simulink model "atril_v2"  (R2019a)
settings: Solver=VariableStepAuto  StartTime=0.0  StopTime=inf  RelTol=1e-3
settings Model: Creator=ASUS  LastModifiedBy=mateo

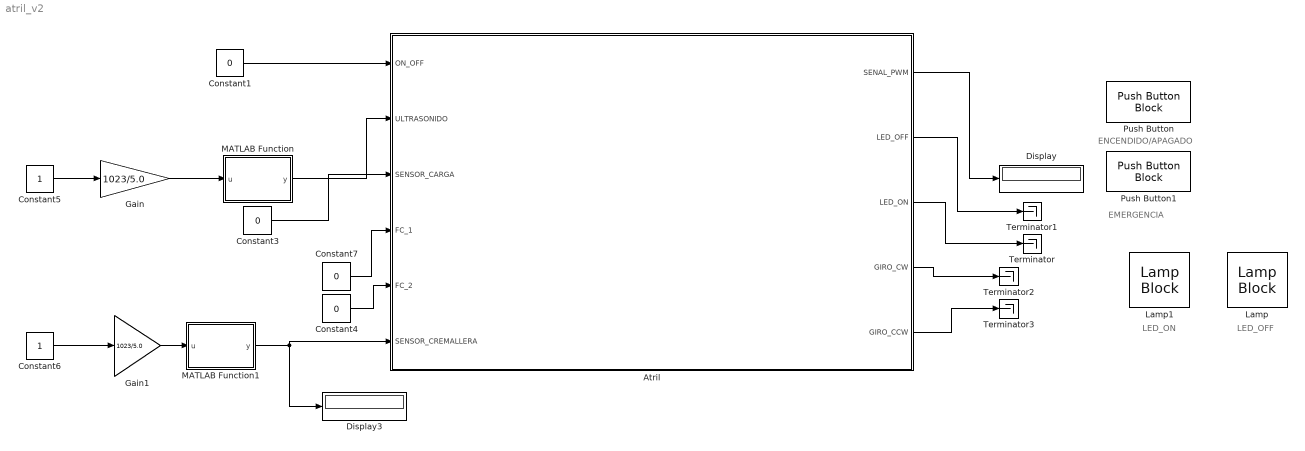
== system atril_v2 ==
  note: LED_OFF
  note: LED_ON
  note: ENCENDIDO/APAGADO
  note: EMERGENCIA
  Atril : Subsystem
  Constant{1,3..4,7} (4 alike) : Constant  Value=0
  Constant5 : Constant
  Constant6 : Constant
  Display : Display
  Display3 : Display
  Gain : Gain  Gain=1023/5.0
  Gain1 : Gain  Gain=1023/5.0
  Lamp : LampBlock  WebBlockId=10
  Lamp1 : LampBlock  WebBlockId=11
  MATLAB Function : MATLAB Function  TreatAsAtomicUnit=on
  MATLAB Function1 : MATLAB Function  TreatAsAtomicUnit=on
  Push Button : PushButtonBlock  WebBlockId=25
  Push Button1 : PushButtonBlock  WebBlockId=26
  Terminator{,1..3} (4 alike) : Terminator
  wires:
  Gain1/1 -> MATLAB Function1/1(u)
  Constant6/1 -> Gain1/1
  Constant5/1 -> Gain/1
  Gain/1 -> MATLAB Function/1(u)
  MATLAB Function1/1(y) -> Atril/6(SENSOR_CREMALLERA), Display3/1
  Constant1/1 -> Atril/1(ON_OFF)
  MATLAB Function/1(y) -> Atril/2(ULTRASONIDO)
  Constant3/1 -> Atril/3(SENSOR_CARGA)
  Constant7/1 -> Atril/4(FC_1)
  Constant4/1 -> Atril/5(FC_2)
  Atril/1(SENAL_PWM) -> Display/1
  Atril/2(LED_OFF) -> Terminator1/1
  Atril/3(LED_ON) -> Terminator/1
  Atril/4(GIRO_CW) -> Terminator2/1
  Atril/5(GIRO_CCW) -> Terminator3/1

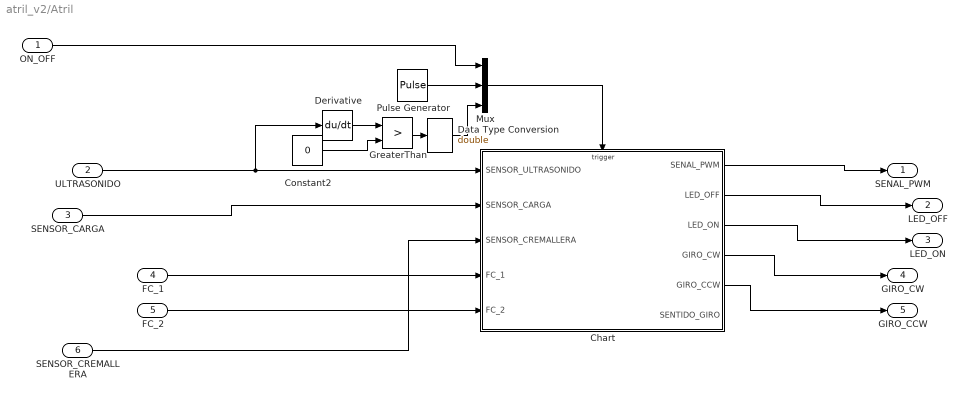
== system atril_v2/Atril ==
  ON_OFF : Inport
  ULTRASONIDO : Inport  Port=2
  SENSOR_CARGA : Inport  Port=3
  FC_1 : Inport  Port=4
  FC_2 : Inport  Port=5
  SENSOR_CREMALLERA : Inport  Port=6
  Chart : Stateflow chart  TreatAsAtomicUnit=on
  Constant2 : Constant  Value=0
  Data Type Conversion : DataTypeConversion  OutDataTypeStr=double
  Derivative : Derivative
  GreaterThan : RelationalOperator  Operator=>  OutDataTypeStr=boolean  RndMeth=Simplest
  Mux : Mux  Inputs=3
  Pulse Generator : DiscretePulseGenerator  PulseType=Time based  Period=10  PulseWidth=0.5
  SENAL_PWM : Outport
  LED_OFF : Outport  Port=2
  LED_ON : Outport  Port=3
  GIRO_CW : Outport  Port=4
  GIRO_CCW : Outport  Port=5
  wires:
  Pulse Generator/1 -> Mux/2
  Constant2/1 -> GreaterThan/2
  ULTRASONIDO/1 -> Chart/1(SENSOR_ULTRASONIDO), Derivative/1
  Mux/1 -> Chart/Trigger
  SENSOR_CREMALLERA/1 -> Chart/3(SENSOR_CREMALLERA)
  SENSOR_CARGA/1 -> Chart/2(SENSOR_CARGA)
  ON_OFF/1 -> Mux/1
  Derivative/1 -> GreaterThan/1
  Chart/1(SENAL_PWM) -> SENAL_PWM/1
  FC_2/1 -> Chart/5(FC_2)
  Chart/2(LED_OFF) -> LED_OFF/1
  FC_1/1 -> Chart/4(FC_1)
  Chart/3(LED_ON) -> LED_ON/1
  Chart/4(GIRO_CW) -> GIRO_CW/1
  Chart/5(GIRO_CCW) -> GIRO_CCW/1
  GreaterThan/1 -> Data Type Conversion/1
  Data Type Conversion/1 -> Mux/3

== matlab function atril_v2/MATLAB Function1 ==
  data: u input; y output
function y = fcn(u)

y = u;

== matlab function atril_v2/MATLAB Function ==
  data: u input; y output
function y = fcn(u)

y = u;

== stateflow chart atril_v2/Atril/Chart ==
  state ESTADO_ON
    state e1
      entry:
      LED_ON=1;
      LED_OFF=0;
      SENAL_PWM=0;
      SENTIDO_GIRO=0;
    state Stand_by
    state e4
      entry:
      SENAL_PWM=0.5;
      GIRO_CW=0;
      GIRO_CCW=1;
    state e2
      entry:
      SENAL_PWM=0.5;
      GIRO_CW=1;
      GIRO_CCW=0;
      FC=SENSOR_ULTRASONIDO*2/1;
    state e3
      entry:
      SENAL_PWM=0;
    (default) -> e1
    e1 -> Stand_by
    Stand_by -> (junction 41) : [SENSOR_ULTRASONIDO>1.4]
    e4 -> e1 : [FC_2==1]
    (junction 41) -> e2 : [SENSOR_CARGA==1]
    e3 -> e4
    e2 -> e3 [order 1] : [SENSOR_CREMALLERA>=FC]
    e2 -> e3 [order 2] : [FC_1==1]
  state EMERGENCIA
    entry:
    LED_ON=0;
    LED_OFF=0;
    SENAL_PWM=0;
    SENTIDO_GIRO=0
  state ESTADO_OFF
    entry:
    LED_ON=0;
    LED_OFF=1;
    SENAL_PWM=0;
    SENTIDO_GIRO=0;
  ESTADO_ON -> EMERGENCIA [order 2] : EMERGENCIA
  EMERGENCIA -> (junction 22) : EMERGENCIA
  ESTADO_OFF -> ESTADO_ON : ON_OFF
  ESTADO_ON -> ESTADO_OFF [order 1] : ON_OFF
  (junction 22) -> ESTADO_OFF
  (default) -> ESTADO_OFF
  data: SENSOR_ULTRASONIDO input; SENSOR_CARGA input; SENSOR_CREMALLERA input; SENAL_PWM output =0; LED_OFF output =0; LED_ON output =0; FC_1 input; FC_2 input; GIRO_CW output =0; GIRO_CCW output =0; SENTIDO_GIRO output; FC local
  events: Clock input EITHER_EDGE_EVENT; ON_OFF input RISING_EDGE_EVENT; EMERGENCIA input FALLING_EDGE_EVENT
